simulink model "Teleoperation_Task_Space"  (R2021b)
settings: Solver=FixedStepAuto  StartTime=0.0  StopTime=20  FixedStep=Ts  RelTol=1e-3
values from neighbouring files (symbols this model uses):
  alphas_m = 25.0 * ones(1,dh.dof)    [setup_teleop.m]
  alphas_s = 16.5 * ones(1,dh.dof)    [setup_teleop.m]
  B_m = diag(ones(1,dh.dof)) * 32    [setup_teleop.m]
  B_s = diag(ones(1,dh.dof)) * 4    [setup_teleop.m]
  fc_in = 0.8    [setup_teleop.m]
  gravity = [0 0 9.81]'    [setup_robot.m]
  K_g = eye(dh.dof) * k_g    [setup_teleop.m]
  K_m = diag(ones(1,dh.dof)) * 22    [setup_teleop.m]
  K_s = diag(ones(1,dh.dof)) * 4    [setup_teleop.m]
  lambdas_m = 7.5 * ones(1,dh.dof)    [setup_teleop.m]
  lambdas_s = 3.0 * ones(1,dh.dof)    [setup_teleop.m]
  M_m = diag(ones(1,dh.dof)) * 22    [setup_teleop.m]
  M_s = diag(ones(1,dh.dof)) * 1    [setup_teleop.m]
  T_m2s = 25 / 1000 / Ts    (= 25)    [setup_teleop.m]
  T_s2m = 25 / 1000 / Ts    (= 25)    [setup_teleop.m]
  zdq_A = [1 3*wc 3*wc^2 wc^3]    [setup_teleop.m]
  zdq_B = [0 0 0 wc^3]    [setup_teleop.m]
undefined symbols (not defined in the file or in its folder): conf, dh, Fm_A, Fm_B, Fs_A, Fs_B, G, sigbuilder_block, x0
libraries: simulink x2, vrlib x2
(part 1 of 2)
settings Model: Creator=eros  LastModifiedBy=Sebastiano
settings SolverCC: AlgebraicLoopSolver=TrustRegion
settings DebuggingCC: SFMachineParentedDataDiag=warning

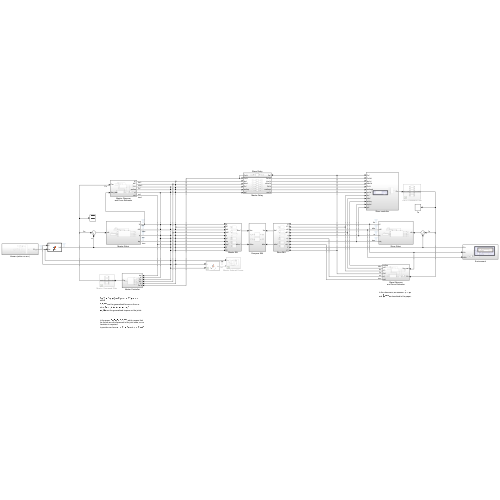
[thumbnail: Simulink's stored preview of the top-level diagram]
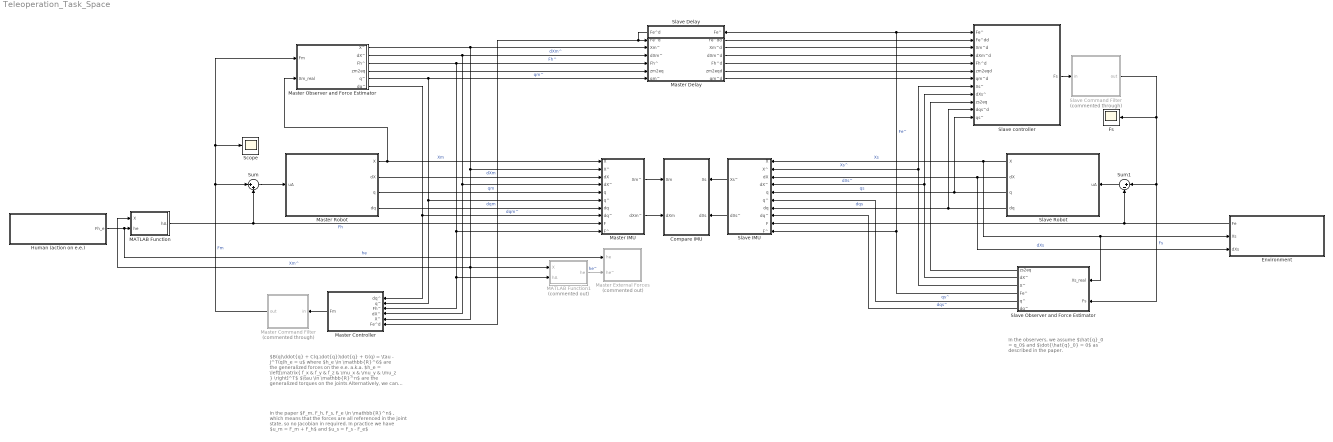
== system Teleoperation_Task_Space ==
  note: In the observers, we assume $\hat{q}_0 = q_0$ and $\dot{\hat{q}_0} = 0$ as described in the paper.
  note: In the paper $F_m, F_h, F_s, F_e \in \mathbb{R}^n$ , which means that the forces are all referenced in the joint state, so no Jacobian in required.
      | In practice we have $u_m = F_m + F_h$ and $u_s = F_s - F_e$
  note: $B(q)\ddot{q} + C(q,\dot{q})\dot{q} + G(q) = \tau - J^T(q)h_e = u$
      | where
      | $h_e \in \mathbb{R}^6$ are the generalized forces on the e.e.
      | a.k.a. $h_e = \left[\matrix{ f_x & f_y & f_z & \mu_x & \mu_y & \mu_z } \right]^T$
      | $\tau \in \mathbb{R}^n$ are the generalized torques on the joints
      |
      | Alternatively, we can write $\tau = J^T(q)\tau_e$ .
  Compare IMU : Subsystem
      settings: PortSchema="{\"entries\":[{\"content\":{\"sides\":[{\"content\":{\"connectorIds\":[\"In1\",\"In2\"]},\"type\":\"ConnectorPlacement.EquallySpacedRectSide\",\"uuid\":\"eee4eb85-6cb8-4462-85fc-1aafb3c3937f\"},{\"content\":{\"connectorIds\":[\"In3\",\"In4\"],\"side\":\"RIGHT\"},\"type\":\"ConnectorPlacement.EquallySpacedRectSide\",\"uuid\":\"5ab37ec6-6ee1-47e9-aff6-41baaee9b59b\"},{\"content\":{\"connectorIds\":[],\"side\":\"TOP\"},\"type\":\"ConnectorPlacement.EquallySpacedRectSide\",\"uuid\":\"6f11ee79-2d90-4b50-8360-b99d360f33b3\"}]},\"type\":\"ConnectorPlacement.EquallySpacedConnector\",\"uuid\":\"5676dc65-12f4-4a54-a0ce-a07c6c462ad2\"}],\"packageUris\":[\"http://schema.mathworks.com/mf0/Connector/R2020b\"],\"version\":\"1.0\"}"
  Environment : Subsystem
      settings: PortSchema="{\"entries\":[{\"content\":{\"sides\":[{\"content\":{\"connectorIds\":[\"Out1\",\"In1\",\"In2\"]},\"type\":\"ConnectorPlacement.EquallySpacedRectSide\",\"uuid\":\"3a683f5f-8229-405f-b97f-b506986b9524\"},{\"content\":{\"connectorIds\":[],\"side\":\"RIGHT\"},\"type\":\"ConnectorPlacement.EquallySpacedRectSide\",\"uuid\":\"ee737040-7d2a-42b5-b72e-c46d7dc1a0a9\"},{\"content\":{\"connectorIds\":[],\"side\":\"TOP\"},\"type\":\"ConnectorPlacement.EquallySpacedRectSide\",\"uuid\":\"297da6e9-ed01-499d-b3c2-0f0e3cad7b3e\"}]},\"type\":\"ConnectorPlacement.EquallySpacedConnector\",\"uuid\":\"c177a36f-944e-4ac9-b62c-2e9de2d24660\"}],\"packageUris\":[\"http://schema.mathworks.com/mf0/Connector/R2020b\"],\"version\":\"1.0\"}"
  Fs : Scope
  Human (action on e.e.) : Subsystem
  MATLAB Function : MATLAB Function  TreatAsAtomicUnit=on
  MATLAB Function1 : MATLAB Function  Commented=on  TreatAsAtomicUnit=on
  Master Command Filter : Subsystem  Commented=through
  Master Controller : Subsystem
  Master Delay : Subsystem
  Master External Forces : Subsystem  Commented=on
  Master IMU : Subsystem
  Master Observer and Force Estimator : Subsystem
  Master Robot : Subsystem
  Scope : Scope
  Slave Command Filter : Subsystem  Commented=through
  Slave Delay : Subsystem
  Slave IMU : Subsystem
  Slave Observer and Force Estimator : Subsystem
  Slave Robot : Subsystem
  Slave controller : Subsystem
  Sum : Sum  Inputs=|++
  Sum1 : Sum  Inputs=|+-
  wires:
  Slave Observer and Force Estimator/5(q^) -> Slave IMU/6(q^)  "qs^"
  Master Controller/1(Fm) -> Master Command Filter/1(in)
  Slave Observer and Force Estimator/1(zs2eq) -> Slave controller/10(zs2eq)
  Master Observer and Force Estimator/1(X^) -> Master Delay/2(Xm^), Master IMU/2(X^), MATLAB Function1/1(X), Master Controller/5(X^), MATLAB Function/1(X)  "Xm^"
  Slave Observer and Force Estimator/4(Fe^) -> Slave controller/1(Fe^), Slave Delay/1(Fe^), Slave IMU/10(F^)  "Fe^"
  Master Observer and Force Estimator/3(Fh^) -> Master Delay/4(Fh^), Master IMU/10(F^), MATLAB Function1/2(hA), Master Controller/3(Fh^)  "Fh^"
  Slave Observer and Force Estimator/6(dq^) -> Slave IMU/8(dq^)  "dqs^"
  Master Observer and Force Estimator/2(dX^) -> Master Delay/3(dXm^), Master IMU/4(dX^), Master Controller/4(dX^)  "dXm^"
  Slave controller/1(Fs) -> Slave Command Filter/1(in)
  Master Command Filter/1(out) -> Scope/1, Master Observer and Force Estimator/1(Fm), Sum/1  "Fm"
  Slave Command Filter/1(out) -> Slave Observer and Force Estimator/2(Fs), Sum1/1, Fs/1  "Fs"
  Master Observer and Force Estimator/4(zm2eq) -> Master Delay/5(zm2eq)
  Master Delay/1(Fe^dd) -> Slave controller/2(Fe^dd)
  Master Delay/3(dXm^d) -> Slave controller/4(dXm^d)
  Master Delay/2(Xm^d) -> Slave controller/3(Xm^d)
  Master Delay/4(Fh^d) -> Slave controller/5(Fh^d)
  Master Delay/5(zm2eqd) -> Slave controller/6(zm2eqd)
  Slave Delay/1(Fe^d) -> Master Controller/6(Fe^d), Master Delay/1(Fe^d)
  Slave Robot/3(q) -> Slave IMU/5(q), Slave controller/12(qs^)  "qs"
  Slave Robot/4(dq) -> Slave IMU/7(dq), Slave controller/11(dqs^d)  "dqs"
  MATLAB Function1/1(he) -> Master External Forces/2(he^)  "he^"
  Human (action on e.e.)/1(Fh_e) -> MATLAB Function/2(he), Master External Forces/1(he)  "he"
  Master Robot/1(X) -> Master Observer and Force Estimator/2(Xm_real), Master IMU/1(X)  "Xm"
  MATLAB Function/1(hA) -> Sum/2, Master IMU/9(F)  "Fh"
  Sum/1 -> Master Robot/1(uA)
  Master Robot/3(q) -> Master IMU/5(q)  "qm"
  Master Observer and Force Estimator/5(q^) -> Master Controller/2(q^), Master IMU/6(q^), Master Delay/6(qm^)  "qm^"
  Master Observer and Force Estimator/6(dq^) -> Master Controller/1(dq^), Master IMU/8(dq^)  "dqm^"
  Master Robot/4(dq) -> Master IMU/7(dq)  "dqm"
  Master Robot/2(dX) -> Master IMU/3(dX)  "dXm"
  Master IMU/2(dXm^) -> Compare IMU/2(dXm)
  Master IMU/1(Xm^) -> Compare IMU/1(Xm)
  Sum1/1 -> Slave Robot/1(uA)
  Slave Robot/1(X) -> Slave Observer and Force Estimator/1(Xs_real), Environment/1(Xs), Slave IMU/1(X)  "Xs"
  Slave Robot/2(dX) -> Environment/2(dXs), Slave IMU/3(dX)  "dXs"
  Slave Observer and Force Estimator/3(X^) -> Slave controller/8(Xs^), Slave IMU/2(X^)  "Xs^"
  Slave Observer and Force Estimator/2(dX^) -> Slave IMU/4(dX^), Slave controller/9(dXs^)  "dXs^"
  Slave IMU/1(Xs^) -> Compare IMU/3(Xs)
  Slave IMU/2(dXs^) -> Compare IMU/4(dXs)
  Master Delay/6(qm^d) -> Slave controller/7(qm^d)
  Environment/1(Fe) -> Sum1/2, Slave IMU/9(F)

== system Teleoperation_Task_Space/Compare IMU ==
  Xm : Inport
  dXm : Inport  Port=2
  Xs : Inport  Port=3
  dXs : Inport  Port=4
  Speed : Subsystem
      settings: PortSchema="{\"entries\":[{\"content\":{\"sides\":[{\"content\":{\"connectorIds\":[\"In1\"]},\"type\":\"ConnectorPlacement.EquallySpacedRectSide\",\"uuid\":\"98f8c5d8-e26e-427c-a81e-60bbe3a3ab4d\"},{\"content\":{\"connectorIds\":[\"In2\"],\"side\":\"RIGHT\"},\"type\":\"ConnectorPlacement.EquallySpacedRectSide\",\"uuid\":\"a51aa647-09cd-4fb3-b31a-f2bc2bc6e0ff\"},{\"content\":{\"connectorIds\":[],\"side\":\"TOP\"},\"type\":\"ConnectorPlacement.EquallySpacedRectSide\",\"uuid\":\"9387bbe5-2fda-43cb-b346-55f243092f42\"}]},\"type\":\"ConnectorPlacement.EquallySpacedConnector\",\"uuid\":\"8debe184-3b59-4f16-84f4-2d6030e17ba5\"}],\"packageUris\":[\"http://schema.mathworks.com/mf0/Connector/R2020b\"],\"version\":\"1.0\"}"
  State : Subsystem
      settings: PortSchema="{\"entries\":[{\"content\":{\"sides\":[{\"content\":{\"connectorIds\":[\"In1\"]},\"type\":\"ConnectorPlacement.EquallySpacedRectSide\",\"uuid\":\"98f8c5d8-e26e-427c-a81e-60bbe3a3ab4d\"},{\"content\":{\"connectorIds\":[\"In2\"],\"side\":\"RIGHT\"},\"type\":\"ConnectorPlacement.EquallySpacedRectSide\",\"uuid\":\"a51aa647-09cd-4fb3-b31a-f2bc2bc6e0ff\"},{\"content\":{\"connectorIds\":[],\"side\":\"TOP\"},\"type\":\"ConnectorPlacement.EquallySpacedRectSide\",\"uuid\":\"9387bbe5-2fda-43cb-b346-55f243092f42\"}]},\"type\":\"ConnectorPlacement.EquallySpacedConnector\",\"uuid\":\"8debe184-3b59-4f16-84f4-2d6030e17ba5\"}],\"packageUris\":[\"http://schema.mathworks.com/mf0/Connector/R2020b\"],\"version\":\"1.0\"}"
  wires:
  Xm/1 -> State/2(q_m)
  Xs/1 -> State/1(q_s)
  dXm/1 -> Speed/1(dq_m)
  dXs/1 -> Speed/2(dq_s)

== system Teleoperation_Task_Space/Environment ==
  note: Spring Environment
  note: Spring-Damper Environment
  Xs : Inport
  dXs : Inport  Port=2
  Constant1 : Constant  Value=[0 0]
  Constant2 : Constant  Value=[0.43 0.41]
  Constant3 : Constant  Value=[0 0]
  Manual Switch : ManualSwitch
  Manual Switch1 : ManualSwitch
  Multiply : Gain  Gain=150*eye(2)  Multiplication=Matrix(K*u)
  Multiply1 : Gain  Gain=10*eye(2)  Multiplication=Matrix(K*u)
  Sum : Sum  Inputs=|++
  Sum2 : Sum  Inputs=+-|
  Fe : Outport
  wires:
  Sum/1 -> Manual Switch/1
  Sum2/1 -> Multiply/1
  Constant2/1 -> Sum2/2
  Xs/1 -> Sum2/1
  Constant1/1 -> Manual Switch1/2
  Manual Switch/1 -> Fe/1
  Multiply/1 -> Sum/1
  Manual Switch1/1 -> Sum/2
  Multiply1/1 -> Manual Switch1/1
  dXs/1 -> Multiply1/1
  Constant3/1 -> Manual Switch/2

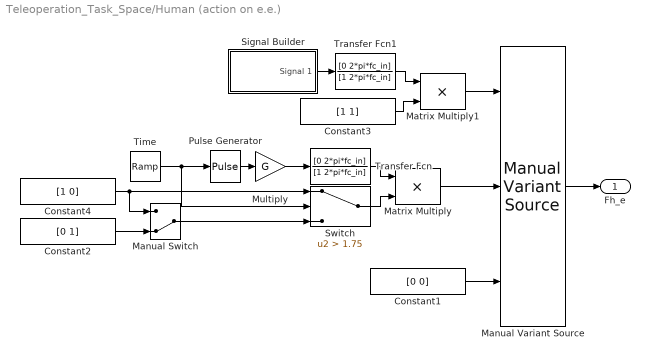
== system Teleoperation_Task_Space/Human (action on e.e.) ==
  Constant1 : Constant  Value=[0 0]
  Constant2 : Constant  Value=[0 1]
  Constant3 : Constant  Value=[1 1]
  Constant4 : Constant  Value=[1 0]
  Manual Variant Source : simulink/Signal Routing/Manual Variant Source  NumChoices=3  LabelModeActiveChoice=V_1
  Manual Switch : ManualSwitch  CurrentSetting=0
  Matrix Multiply : Product
  Matrix Multiply1 : Product
  Multiply : Gain  Gain=G
  Pulse Generator : DiscretePulseGenerator  PulseType=Time based  TimeSource=Use external signal  Period=10  PulseWidth=5  PhaseDelay=0.5
  Signal Builder : Subsystem  Tag=STV Subsys  LoadFcn=sigbuilder_block('load');  StartFcn=sigbuilder_block('start');  StopFcn=sigbuilder_block('stop');  ClipboardFcn=sigbuilder_block('clipboard');  mask(Sigbuilder block){tuvar=[0:10]}
      mask help: Simulink:masks:SigbuilderBlock_MD
      mask init:
      | if ~strcmp(get_param(bdroot(gcbh),'SimulationStatus'),'stopped') tuvar = sigbuilder_block('maskInit'); end
      settings: CopyFcn=sigbuilder_block('copy');  DeleteFcn=sigbuilder_block('delete');  ModelCloseFcn=sigbuilder_block('modelClose');  PreSaveFcn=sigbuilder_block('preSave');  PauseFcn=sigbuilder_block('pause');  ContinueFcn=sigbuilder_block('continue');  NameChangeFcn=sigbuilder_block('namechange');  OpenFcn=sigbuilder_block('open',[47.25 0 1392.75 752.25 ]);  CloseFcn=sigbuilder_block('close');
      mask Display: plot(0, 0, 100, 100,[2, 2, 32, 32, 2], [68, 8, 8, 68, 68],[32, 2], [38, 38], [32, 19, 2],[53, 60, 44], [32, 17, 17, 2],[16, 16, 31, 31]);txt = getActiveGroup(gcbh);text(2, 100, txt,'verticalAlignment', 'top');
  Switch : Switch  Criteria=u2 > Threshold  Threshold=1.75
  Time : simulink/Sources/Ramp  slope=1  start=0  InitialOutput=0
  Transfer Fcn : TransferFcn  Numerator=[0 2*pi*fc_in]  Denominator=[1 2*pi*fc_in]
  Transfer Fcn1 : TransferFcn  Numerator=[0 2*pi*fc_in]  Denominator=[1 2*pi*fc_in]
  Fh_e : Outport
  wires:
  Switch/1 -> Matrix Multiply/2
  Constant2/1 -> Manual Switch/2
  Transfer Fcn/1 -> Matrix Multiply/1
  Time/1 -> Switch/2, Pulse Generator/1
  Constant4/1 -> Manual Switch/1, Switch/1
  Manual Switch/1 -> Switch/3
  Matrix Multiply/1 -> Manual Variant Source/2
  Constant1/1 -> Manual Variant Source/3
  Signal Builder/1(Signal 1) -> Transfer Fcn1/1
  Pulse Generator/1 -> Multiply/1
  Multiply/1 -> Transfer Fcn/1
  Transfer Fcn1/1 -> Matrix Multiply1/1
  Constant3/1 -> Matrix Multiply1/2
  Matrix Multiply1/1 -> Manual Variant Source/1
  Manual Variant Source/1 -> Fh_e/1

== system Teleoperation_Task_Space/Master Command Filter ==
  in : Inport
  Demux : Demux  Outputs=6
  Filter{,1..5} (6 alike) : TransferFcn  Numerator=Fm_B  Denominator=Fm_A
  Mux : Mux  Inputs=6
  out : Outport
  wires:
  Demux/4 -> Filter3/1
  Demux/6 -> Filter5/1
  Demux/2 -> Filter1/1
  Demux/5 -> Filter4/1
  Demux/1 -> Filter/1
  Demux/3 -> Filter2/1
  in/1 -> Demux/1
  Mux/1 -> out/1
  Filter/1 -> Mux/1
  Filter1/1 -> Mux/2
  Filter2/1 -> Mux/3
  Filter3/1 -> Mux/4
  Filter4/1 -> Mux/5
  Filter5/1 -> Mux/6

== system Teleoperation_Task_Space/Master Controller ==
  note: Here we provide q^ and dq^ just to avoid calculating them
  dq^ : Inport
  q^ : Inport  Port=2
  Fh^ : Inport  Port=3
  dX^ : Inport  Port=4
  X^ : Inport  Port=5
  Fe^d : Inport  Port=6
  Master Controller : MATLAB Function  TreatAsAtomicUnit=on
  Fm : Outport
  wires:
  Fh^/1 -> Master Controller/5(Fh)
  Fe^d/1 -> Master Controller/6(Fe_d)
  Master Controller/1(Fm) -> Fm/1  "Fm"
  X^/1 -> Master Controller/3(Xm)
  dX^/1 -> Master Controller/4(dXm)
  dq^/1 -> Master Controller/2(dqm)
  q^/1 -> Master Controller/1(qm)

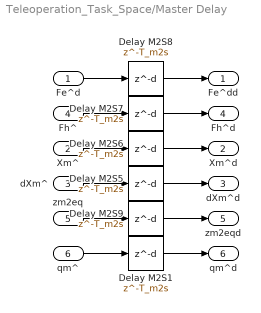
== system Teleoperation_Task_Space/Master Delay ==
  Fe^d : Inport
  Xm^ : Inport  Port=2
  dXm^ : Inport  Port=3
  Fh^ : Inport  Port=4
  zm2eq : Inport  Port=5
  qm^ : Inport  Port=6
  Delay M2S{1,5..9} (6 alike) : Delay  DelayLength=T_m2s
  Fe^dd : Outport
  Xm^d : Outport  Port=2
  dXm^d : Outport  Port=3
  Fh^d : Outport  Port=4
  zm2eqd : Outport  Port=5
  qm^d : Outport  Port=6
  wires:
  zm2eq/1 -> Delay M2S9/1
  Delay M2S6/1 -> Xm^d/1
  dXm^/1 -> Delay M2S5/1
  Fe^d/1 -> Delay M2S8/1
  Fh^/1 -> Delay M2S7/1
  Delay M2S5/1 -> dXm^d/1
  Delay M2S7/1 -> Fh^d/1
  Xm^/1 -> Delay M2S6/1
  Delay M2S8/1 -> Fe^dd/1
  Delay M2S9/1 -> zm2eqd/1
  Delay M2S1/1 -> qm^d/1
  qm^/1 -> Delay M2S1/1

== system Teleoperation_Task_Space/Master External Forces ==
  he : Inport
  he^ : Inport  Port=2
  Master he : Scope  NumInputPorts=2
  Mux : Mux  Inputs=2
  Mux1 : Mux  Inputs=2
  qm : Demux  Outputs=dh.dof
  qs : Demux  Outputs=dh.dof
  wires:
  he/1 -> qm/1
  he^/1 -> qs/1
  qm/1 -> Mux/1
  qs/1 -> Mux/2
  qm/2 -> Mux1/1
  qs/2 -> Mux1/2
  Mux/1 -> Master he/1
  Mux1/1 -> Master he/2

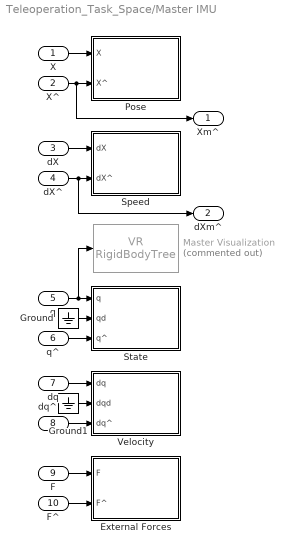
== system Teleoperation_Task_Space/Master IMU ==
  X : Inport
  X^ : Inport  Port=2
  dX : Inport  Port=3
  dX^ : Inport  Port=4
  q : Inport  Port=5
  q^ : Inport  Port=6
  dq : Inport  Port=7
  dq^ : Inport  Port=8
  F : Inport  Port=9
  F^ : Inport  Port=10
  External Forces : Subsystem
  Ground : Ground
  Ground1 : Ground
  Master Visualization : vrlib/VR RigidBodyTree  Commented=on  RBT=UR5_robot  useRBT=on  Ts=-1  ForceViewerOpen=on
      settings: SourceProductBaseCode=SL
  Pose : Subsystem
  Speed : Subsystem
  State : Subsystem
  Velocity : Subsystem
  Xm^ : Outport
  dXm^ : Outport  Port=2
  wires:
  q/1 -> Master Visualization/1, State/1(q)
  q^/1 -> State/3(q^)
  F/1 -> External Forces/1(F)
  dq/1 -> Velocity/1(dq)
  F^/1 -> External Forces/2(F^)
  dq^/1 -> Velocity/3(dq^)
  Ground/1 -> State/2(qd)
  Ground1/1 -> Velocity/2(dqd)
  X^/1 -> Xm^/1, Pose/2(X^)
  X/1 -> Pose/1(X)
  dX/1 -> Speed/1(dX)
  dX^/1 -> dXm^/1, Speed/2(dX^)

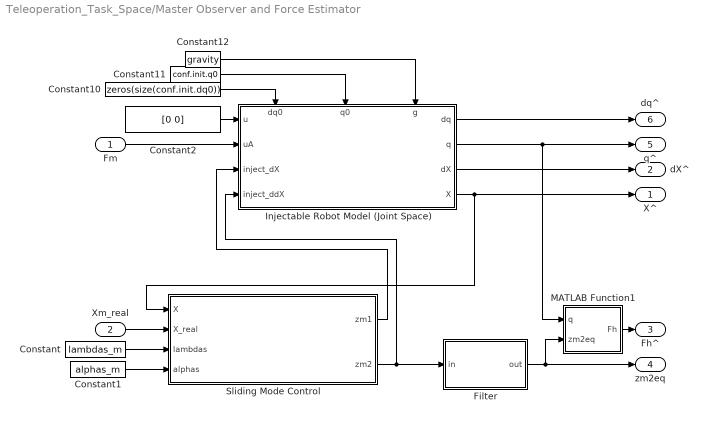
== system Teleoperation_Task_Space/Master Observer and Force Estimator ==
  Fm : Inport
  Xm_real : Inport  Port=2
  Constant : Constant  Value=lambdas_m
  Constant1 : Constant  Value=alphas_m
  Constant10 : Constant  Value=zeros(size(conf.init.dq0))
  Constant11 : Constant  Value=conf.init.q0
  Constant12 : Constant  Value=gravity
  Constant2 : Constant  Value=[0 0]
  Filter : Subsystem
  Injectable Robot Model (Joint Space) : Subsystem
      settings: PortSchema="{\"entries\":[{\"content\":{\"sides\":[{\"content\":{\"connectorIds\":[\"In1\",\"In2\",\"In3\",\"In4\"]},\"type\":\"ConnectorPlacement.EquallySpacedRectSide\",\"uuid\":\"a8701c64-329e-4144-b882-ecf5d621aff2\"},{\"content\":{\"connectorIds\":[\"Out1\",\"Out2\",\"Out3\",\"Out4\"],\"side\":\"RIGHT\"},\"type\":\"ConnectorPlacement.EquallySpacedRectSide\",\"uuid\":\"4e168703-1cb9-438c-bc6b-9b2d7fbb809e\"},{\"content\":{\"connectorIds\":[\"In5\",\"In6\",\"In7\"],\"side\":\"TOP\"},\"type\":\"ConnectorPlacement.EquallySpacedRectSide\",\"uuid\":\"8fbcb29e-7fab-4224-b4ad-ee01c13d675a\"}]},\"type\":\"ConnectorPlacement.EquallySpacedConnector\",\"uuid\":\"fa721fab-1ce6-4fdf-95fa-8ada3ed2d65c\"}],\"packageUris\":[\"http://schema.mathworks.com/mf0/Connector/R2020b\"],\"version\":\"1.0\"}"
  MATLAB Function1 : MATLAB Function  TreatAsAtomicUnit=on
  Sliding Mode Control : Subsystem
  X^ : Outport
  dX^ : Outport  Port=2
  Fh^ : Outport  Port=3
  zm2eq : Outport  Port=4
  q^ : Outport  Port=5
  dq^ : Outport  Port=6
  wires:
  Filter/1(out) -> MATLAB Function1/2(zm2eq), zm2eq/1
  Sliding Mode Control/1(zm1) -> Injectable Robot Model (Joint Space)/3(inject_dX)
  Sliding Mode Control/2(zm2) -> Injectable Robot Model (Joint Space)/4(inject_ddX), Filter/1(in)
  Constant1/1 -> Sliding Mode Control/4(alphas)
  Constant/1 -> Sliding Mode Control/3(lambdas)
  Xm_real/1 -> Sliding Mode Control/2(X_real)
  Injectable Robot Model (Joint Space)/4(X) -> X^/1, Sliding Mode Control/1(X)
  Injectable Robot Model (Joint Space)/3(dX) -> dX^/1
  Constant11/1 -> Injectable Robot Model (Joint Space)/6(q0)
  Constant10/1 -> Injectable Robot Model (Joint Space)/5(dq0)
  Injectable Robot Model (Joint Space)/1(dq) -> dq^/1
  Constant12/1 -> Injectable Robot Model (Joint Space)/7(g)
  Injectable Robot Model (Joint Space)/2(q) -> MATLAB Function1/1(q), q^/1
  MATLAB Function1/1(Fh) -> Fh^/1
  Constant2/1 -> Injectable Robot Model (Joint Space)/1(u)
  Fm/1 -> Injectable Robot Model (Joint Space)/2(uA)

== system Teleoperation_Task_Space/Master Robot ==
  uA : Inport
  Constant10 : Constant  Value=conf.init.dq0
  Constant11 : Constant  Value=conf.init.q0
  Constant12 : Constant  Value=gravity
  Constant3 : Constant  Value=[0 0]
  Injectable Robot Model (Joint Space) : Subsystem
      settings: PortSchema="{\"entries\":[{\"content\":{\"sides\":[{\"content\":{\"connectorIds\":[\"In1\",\"In2\",\"In3\",\"In4\"]},\"type\":\"ConnectorPlacement.EquallySpacedRectSide\",\"uuid\":\"a8701c64-329e-4144-b882-ecf5d621aff2\"},{\"content\":{\"connectorIds\":[\"Out1\",\"Out2\",\"Out3\",\"Out4\"],\"side\":\"RIGHT\"},\"type\":\"ConnectorPlacement.EquallySpacedRectSide\",\"uuid\":\"4e168703-1cb9-438c-bc6b-9b2d7fbb809e\"},{\"content\":{\"connectorIds\":[\"In5\",\"In6\",\"In7\"],\"side\":\"TOP\"},\"type\":\"ConnectorPlacement.EquallySpacedRectSide\",\"uuid\":\"8fbcb29e-7fab-4224-b4ad-ee01c13d675a\"}]},\"type\":\"ConnectorPlacement.EquallySpacedConnector\",\"uuid\":\"fa721fab-1ce6-4fdf-95fa-8ada3ed2d65c\"}],\"packageUris\":[\"http://schema.mathworks.com/mf0/Connector/R2020b\"],\"version\":\"1.0\"}"
  X : Outport
  dX : Outport  Port=2
  q : Outport  Port=3
  dq : Outport  Port=4
  wires:
  Constant10/1 -> Injectable Robot Model (Joint Space)/5(dq0)
  Constant3/1 -> Injectable Robot Model (Joint Space)/1(u), Injectable Robot Model (Joint Space)/4(inject_ddX), Injectable Robot Model (Joint Space)/3(inject_dX)
  Constant11/1 -> Injectable Robot Model (Joint Space)/6(q0)
  Injectable Robot Model (Joint Space)/2(q) -> q/1
  Injectable Robot Model (Joint Space)/3(dX) -> dX/1
  Constant12/1 -> Injectable Robot Model (Joint Space)/7(g)
  Injectable Robot Model (Joint Space)/4(X) -> X/1
  Injectable Robot Model (Joint Space)/1(dq) -> dq/1
  uA/1 -> Injectable Robot Model (Joint Space)/2(uA)

== system Teleoperation_Task_Space/Slave Command Filter ==
  in : Inport
  Demux : Demux  Outputs=6
  Filter{,1..5} (6 alike) : TransferFcn  Numerator=Fs_B  Denominator=Fs_A
  Mux : Mux  Inputs=6
  out : Outport
  wires:
  Demux/4 -> Filter3/1
  Demux/6 -> Filter5/1
  Demux/2 -> Filter1/1
  Demux/5 -> Filter4/1
  Demux/1 -> Filter/1
  Demux/3 -> Filter2/1
  in/1 -> Demux/1
  Mux/1 -> out/1
  Filter/1 -> Mux/1
  Filter2/1 -> Mux/3
  Filter3/1 -> Mux/4
  Filter4/1 -> Mux/5
  Filter5/1 -> Mux/6
  Filter1/1 -> Mux/2

== system Teleoperation_Task_Space/Slave Delay ==
  Fe^ : Inport
  Delay S2M1 : Delay  DelayLength=T_s2m
  Fe^d : Outport
  wires:
  Delay S2M1/1 -> Fe^d/1
  Fe^/1 -> Delay S2M1/1

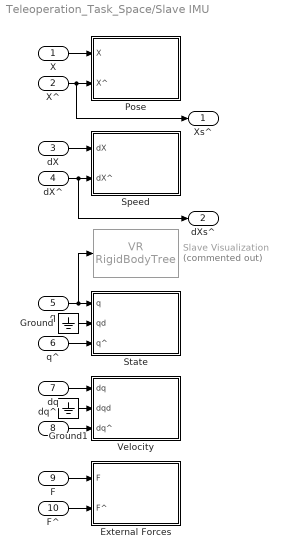
== system Teleoperation_Task_Space/Slave IMU ==
  X : Inport
  X^ : Inport  Port=2
  dX : Inport  Port=3
  dX^ : Inport  Port=4
  q : Inport  Port=5
  q^ : Inport  Port=6
  dq : Inport  Port=7
  dq^ : Inport  Port=8
  F : Inport  Port=9
  F^ : Inport  Port=10
  External Forces : Subsystem
  Ground : Ground
  Ground1 : Ground
  Pose : Subsystem
  Slave Visualization : vrlib/VR RigidBodyTree  Commented=on  RBT=UR5_robot  useRBT=on  Ts=-1  ForceViewerOpen=on
      settings: SourceProductBaseCode=SL
  Speed : Subsystem
  State : Subsystem
  Velocity : Subsystem
  Xs^ : Outport
  dXs^ : Outport  Port=2
  wires:
  q/1 -> Slave Visualization/1, State/1(q)
  q^/1 -> State/3(q^)
  F/1 -> External Forces/1(F)
  dq/1 -> Velocity/1(dq)
  F^/1 -> External Forces/2(F^)
  dq^/1 -> Velocity/3(dq^)
  Ground/1 -> State/2(qd)
  Ground1/1 -> Velocity/2(dqd)
  X^/1 -> Xs^/1, Pose/2(X^)
  X/1 -> Pose/1(X)
  dX/1 -> Speed/1(dX)
  dX^/1 -> dXs^/1, Speed/2(dX^)

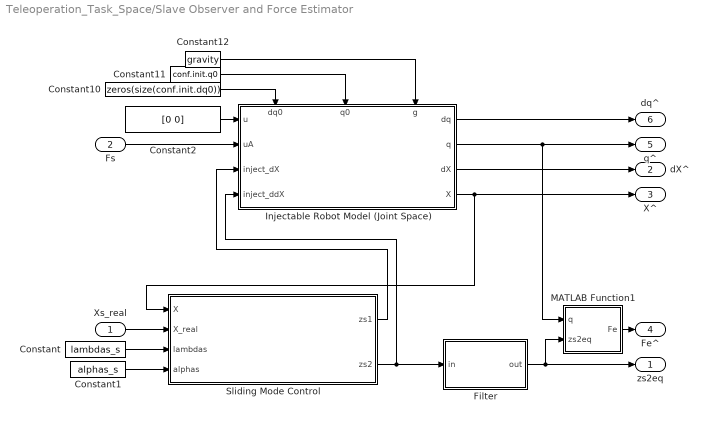
== system Teleoperation_Task_Space/Slave Observer and Force Estimator ==
  Xs_real : Inport
  Fs : Inport  Port=2
  Constant : Constant  Value=lambdas_s
  Constant1 : Constant  Value=alphas_s
  Constant10 : Constant  Value=zeros(size(conf.init.dq0))
  Constant11 : Constant  Value=conf.init.q0
  Constant12 : Constant  Value=gravity
  Constant2 : Constant  Value=[0 0]
  Filter : Subsystem
  Injectable Robot Model (Joint Space) : Subsystem
      settings: PortSchema="{\"entries\":[{\"content\":{\"sides\":[{\"content\":{\"connectorIds\":[\"In1\",\"In2\",\"In3\",\"In4\"]},\"type\":\"ConnectorPlacement.EquallySpacedRectSide\",\"uuid\":\"a8701c64-329e-4144-b882-ecf5d621aff2\"},{\"content\":{\"connectorIds\":[\"Out1\",\"Out2\",\"Out3\",\"Out4\"],\"side\":\"RIGHT\"},\"type\":\"ConnectorPlacement.EquallySpacedRectSide\",\"uuid\":\"4e168703-1cb9-438c-bc6b-9b2d7fbb809e\"},{\"content\":{\"connectorIds\":[\"In5\",\"In6\",\"In7\"],\"side\":\"TOP\"},\"type\":\"ConnectorPlacement.EquallySpacedRectSide\",\"uuid\":\"8fbcb29e-7fab-4224-b4ad-ee01c13d675a\"}]},\"type\":\"ConnectorPlacement.EquallySpacedConnector\",\"uuid\":\"fa721fab-1ce6-4fdf-95fa-8ada3ed2d65c\"}],\"packageUris\":[\"http://schema.mathworks.com/mf0/Connector/R2020b\"],\"version\":\"1.0\"}"
  MATLAB Function1 : MATLAB Function  TreatAsAtomicUnit=on
  Sliding Mode Control : Subsystem
  zs2eq : Outport
  dX^ : Outport  Port=2
  X^ : Outport  Port=3
  Fe^ : Outport  Port=4
  q^ : Outport  Port=5
  dq^ : Outport  Port=6
  wires:
  Filter/1(out) -> MATLAB Function1/2(zs2eq), zs2eq/1
  Sliding Mode Control/1(zs1) -> Injectable Robot Model (Joint Space)/3(inject_dX)
  Sliding Mode Control/2(zs2) -> Injectable Robot Model (Joint Space)/4(inject_ddX), Filter/1(in)
  Constant1/1 -> Sliding Mode Control/4(alphas)
  Constant/1 -> Sliding Mode Control/3(lambdas)
  Xs_real/1 -> Sliding Mode Control/2(X_real)
  Injectable Robot Model (Joint Space)/4(X) -> X^/1, Sliding Mode Control/1(X)
  Injectable Robot Model (Joint Space)/3(dX) -> dX^/1
  Constant11/1 -> Injectable Robot Model (Joint Space)/6(q0)
  Constant10/1 -> Injectable Robot Model (Joint Space)/5(dq0)
  Injectable Robot Model (Joint Space)/1(dq) -> dq^/1
  Constant12/1 -> Injectable Robot Model (Joint Space)/7(g)
  Injectable Robot Model (Joint Space)/2(q) -> MATLAB Function1/1(q), q^/1
  MATLAB Function1/1(Fe) -> Fe^/1
  Constant2/1 -> Injectable Robot Model (Joint Space)/1(u)
  Fs/1 -> Injectable Robot Model (Joint Space)/2(uA)

== system Teleoperation_Task_Space/Slave Robot ==
  uA : Inport
  Constant10 : Constant  Value=conf.init.dq0
  Constant11 : Constant  Value=conf.init.q0
  Constant12 : Constant  Value=gravity
  Constant3 : Constant  Value=[0 0]
  Injectable Robot Model (Joint Space) : Subsystem
      settings: PortSchema="{\"entries\":[{\"content\":{\"sides\":[{\"content\":{\"connectorIds\":[\"In1\",\"In2\",\"In3\",\"In4\"]},\"type\":\"ConnectorPlacement.EquallySpacedRectSide\",\"uuid\":\"a8701c64-329e-4144-b882-ecf5d621aff2\"},{\"content\":{\"connectorIds\":[\"Out1\",\"Out2\",\"Out3\",\"Out4\"],\"side\":\"RIGHT\"},\"type\":\"ConnectorPlacement.EquallySpacedRectSide\",\"uuid\":\"4e168703-1cb9-438c-bc6b-9b2d7fbb809e\"},{\"content\":{\"connectorIds\":[\"In5\",\"In6\",\"In7\"],\"side\":\"TOP\"},\"type\":\"ConnectorPlacement.EquallySpacedRectSide\",\"uuid\":\"8fbcb29e-7fab-4224-b4ad-ee01c13d675a\"}]},\"type\":\"ConnectorPlacement.EquallySpacedConnector\",\"uuid\":\"fa721fab-1ce6-4fdf-95fa-8ada3ed2d65c\"}],\"packageUris\":[\"http://schema.mathworks.com/mf0/Connector/R2020b\"],\"version\":\"1.0\"}"
  X : Outport
  dX : Outport  Port=2
  q : Outport  Port=3
  dq : Outport  Port=4
  wires:
  Constant10/1 -> Injectable Robot Model (Joint Space)/5(dq0)
  Constant3/1 -> Injectable Robot Model (Joint Space)/1(u), Injectable Robot Model (Joint Space)/4(inject_ddX), Injectable Robot Model (Joint Space)/3(inject_dX)
  Constant11/1 -> Injectable Robot Model (Joint Space)/6(q0)
  Injectable Robot Model (Joint Space)/2(q) -> q/1
  Injectable Robot Model (Joint Space)/3(dX) -> dX/1
  Constant12/1 -> Injectable Robot Model (Joint Space)/7(g)
  Injectable Robot Model (Joint Space)/4(X) -> X/1
  Injectable Robot Model (Joint Space)/1(dq) -> dq/1
  uA/1 -> Injectable Robot Model (Joint Space)/2(uA)

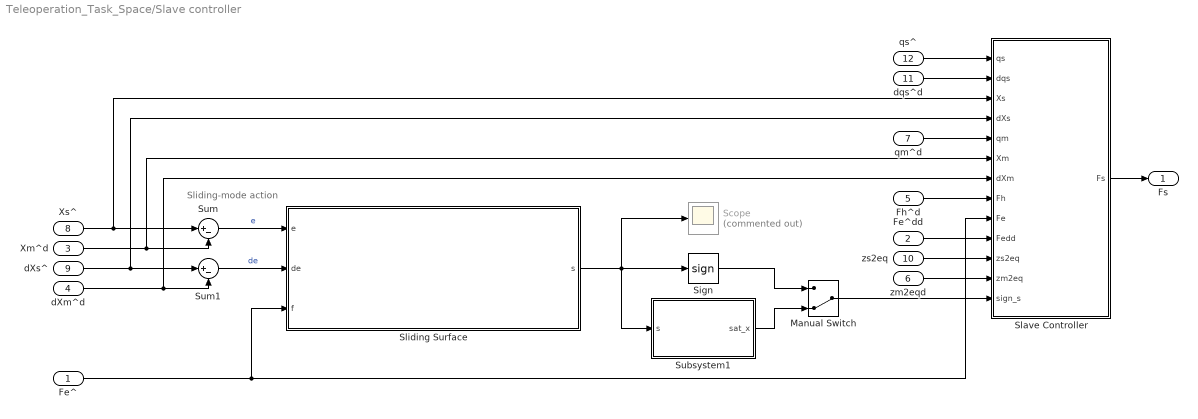
== system Teleoperation_Task_Space/Slave controller ==
  note: Sliding-mode action
  Fe^ : Inport
  Fe^dd : Inport  Port=2
  Xm^d : Inport  Port=3
  dXm^d : Inport  Port=4
  Fh^d : Inport  Port=5
  zm2eqd : Inport  Port=6
  qm^d : Inport  Port=7
  Xs^ : Inport  Port=8
  dXs^ : Inport  Port=9
  zs2eq : Inport  Port=10
  dqs^d : Inport  Port=11
  qs^ : Inport  Port=12
  Manual Switch : ManualSwitch  CurrentSetting=0
  Scope : Scope  Commented=on
  Sign : Signum
  Slave Controller : MATLAB Function  TreatAsAtomicUnit=on
  Sliding Surface : Subsystem
  Subsystem1 : Subsystem
  Sum : Sum  Inputs=|+-
  Sum1 : Sum  Inputs=|+-
  Fs : Outport
  wires:
  zs2eq/1 -> Slave Controller/11(zs2eq)
  Fh^d/1 -> Slave Controller/8(Fh)
  Slave Controller/1(Fs) -> Fs/1
  zm2eqd/1 -> Slave Controller/12(zm2eq)
  Fe^dd/1 -> Slave Controller/10(Fedd)
  Xs^/1 -> Sum/1, Slave Controller/3(Xs)
  Xm^d/1 -> Sum/2, Slave Controller/6(Xm)
  dXs^/1 -> Sum1/1, Slave Controller/4(dXs)
  dXm^d/1 -> Slave Controller/7(dXm), Sum1/2
  Fe^/1 -> Slave Controller/9(Fe), Sliding Surface/3(f)
  Sign/1 -> Manual Switch/1
  Sum/1 -> Sliding Surface/1(e)  "e"
  Sum1/1 -> Sliding Surface/2(de)  "de"
  Sliding Surface/1(s) -> Sign/1, Scope/1, Subsystem1/1(s)
  Subsystem1/1(sat_x) -> Manual Switch/2
  Manual Switch/1 -> Slave Controller/13(sign_s)
  qs^/1 -> Slave Controller/1(qs)
  dqs^d/1 -> Slave Controller/2(dqs)
  qm^d/1 -> Slave Controller/5(qm)

== system Teleoperation_Task_Space/Compare IMU/Speed ==
  dq_m : Inport
  dq_s : Inport  Port=2
  Compare Speed : Scope  NumInputPorts=2
  Mux : Mux  Inputs=2
  Mux1 : Mux  Inputs=2
  qm : Demux  Outputs=dh.dof
  qs : Demux  Outputs=dh.dof
  wires:
  dq_m/1 -> qm/1
  dq_s/1 -> qs/1
  qm/1 -> Mux/1
  qs/1 -> Mux/2
  qm/2 -> Mux1/1
  qs/2 -> Mux1/2
  Mux/1 -> Compare Speed/1
  Mux1/1 -> Compare Speed/2

== system Teleoperation_Task_Space/Compare IMU/State ==
  q_s : Inport
  q_m : Inport  Port=2
  Compare State : Scope  NumInputPorts=2
  Mux : Mux  Inputs=2
  Mux1 : Mux  Inputs=2
  qm : Demux  Outputs=dh.dof
  qs : Demux  Outputs=dh.dof
  wires:
  q_m/1 -> qm/1
  q_s/1 -> qs/1
  qm/1 -> Mux/1
  qs/1 -> Mux/2
  qm/2 -> Mux1/1
  qs/2 -> Mux1/2
  Mux/1 -> Compare State/1
  Mux1/1 -> Compare State/2

== system Teleoperation_Task_Space/Human (action on e.e.)/Signal Builder ==
  Demux : Demux  Tag=STV Demux  Outputs=1
      settings: DisplayOption=none
  FromWs : FromWorkspace  Tag=STV FromWs  VariableName=tuvar
      SigBuilderData=|
      | common.afterFinalStr = 'Extrapolate'
      | common.sampleTime = 0
      | dataSet.timeRange = [0 20]
      | dataSet.name = 'Group 1'
      | sbobj.Groups.Name = 'Group 1'
      | sbobj.Groups.Signals.Name = 'Signal 1'
      | sbobj.Groups.Signals.XData = [0 5 5 10 10 15 15 20]
      | sbobj.Groups.Signals.YData = [10 10 5 5 10 10 5 5]
      | sbobj.Groups.TimeRange = [0 20]
  Signal 1 : Outport  Tag=STV Outport
  wires:
  Demux/1 -> Signal 1/1
  FromWs/1 -> Demux/1

== system Teleoperation_Task_Space/Master IMU/External Forces ==
  F : Inport
  F^ : Inport  Port=2
  Master Fe : Scope  NumInputPorts=2
  Mux : Mux  Inputs=2
  Mux1 : Mux  Inputs=2
  qm : Demux  Outputs=dh.dof
  qs : Demux  Outputs=dh.dof
  wires:
  F/1 -> qm/1
  F^/1 -> qs/1
  qm/1 -> Mux/1
  qs/1 -> Mux/2
  qm/2 -> Mux1/1
  qs/2 -> Mux1/2
  Mux/1 -> Master Fe/1
  Mux1/1 -> Master Fe/2

== system Teleoperation_Task_Space/Master IMU/Pose ==
  X : Inport
  X^ : Inport  Port=2
  Master Pose : Scope  NumInputPorts=2
  Mux : Mux  Inputs=2
  Mux1 : Mux  Inputs=2
  qm : Demux  Outputs=dh.dof
  qm1 : Demux  Outputs=dh.dof
  wires:
  X/1 -> qm/1
  qm/1 -> Mux/1
  qm/2 -> Mux1/1
  Mux/1 -> Master Pose/1
  Mux1/1 -> Master Pose/2
  qm1/2 -> Mux1/2
  X^/1 -> qm1/1
  qm1/1 -> Mux/2

== system Teleoperation_Task_Space/Master IMU/Speed ==
  dX : Inport
  dX^ : Inport  Port=2
  Master Speed : Scope  NumInputPorts=2
  Mux : Mux  Inputs=2
  Mux1 : Mux  Inputs=2
  qm : Demux  Outputs=dh.dof
  qm1 : Demux  Outputs=dh.dof
  wires:
  dX/1 -> qm/1
  qm/1 -> Mux/1
  qm/2 -> Mux1/1
  Mux/1 -> Master Speed/1
  Mux1/1 -> Master Speed/2
  qm1/2 -> Mux1/2
  dX^/1 -> qm1/1
  qm1/1 -> Mux/2

== system Teleoperation_Task_Space/Master IMU/State ==
  q : Inport
  qd : Inport  Port=2
  q^ : Inport  Port=3
  Master State : Scope  NumInputPorts=2
  Mux : Mux  Inputs=3
  Mux1 : Mux  Inputs=3
  qm : Demux  Outputs=dh.dof
  qm1 : Demux  Outputs=dh.dof
  qs : Demux  Outputs=dh.dof
  wires:
  q/1 -> qm/1
  qd/1 -> qs/1
  qm/1 -> Mux/1
  qs/1 -> Mux/2
  qm/2 -> Mux1/1
  qs/2 -> Mux1/2
  Mux/1 -> Master State/1
  Mux1/1 -> Master State/2
  qm1/2 -> Mux1/3
  q^/1 -> qm1/1
  qm1/1 -> Mux/3

== system Teleoperation_Task_Space/Master IMU/Velocity ==
  dq : Inport
  dqd : Inport  Port=2
  dq^ : Inport  Port=3
  Master Velocity : Scope  NumInputPorts=2
  Mux : Mux  Inputs=3
  Mux1 : Mux  Inputs=3
  qm : Demux  Outputs=dh.dof
  qm1 : Demux  Outputs=dh.dof
  qs : Demux  Outputs=dh.dof
  wires:
  dq/1 -> qm/1
  dqd/1 -> qs/1
  qm/1 -> Mux/1
  qs/1 -> Mux/2
  qm/2 -> Mux1/1
  qs/2 -> Mux1/2
  Mux/1 -> Master Velocity/1
  Mux1/1 -> Master Velocity/2
  qm1/2 -> Mux1/3
  dq^/1 -> qm1/1
  qm1/1 -> Mux/3

== system Teleoperation_Task_Space/Master Observer and Force Estimator/Filter ==
  in : Inport
  Demux : Demux  Outputs=2
  Filter : TransferFcn  Numerator=zdq_B  Denominator=zdq_A
  Filter1 : TransferFcn  Numerator=zdq_B  Denominator=zdq_A
  Mux : Mux  Inputs=2
  out : Outport
  wires:
  Demux/2 -> Filter1/1
  Demux/1 -> Filter/1
  in/1 -> Demux/1
  Mux/1 -> out/1
  Filter/1 -> Mux/1
  Filter1/1 -> Mux/2

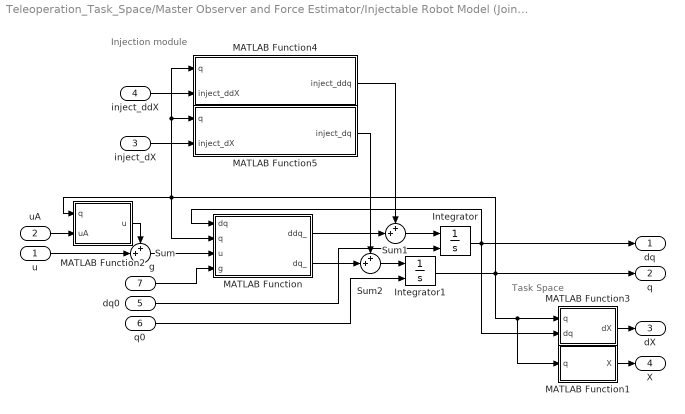
== system Teleoperation_Task_Space/Master Observer and Force Estimator/Injectable Robot Model (Joint Space) ==
  note: Injection module
  note: Task Space
  u : Inport
  uA : Inport  Port=2
  inject_dX : Inport  Port=3
  inject_ddX : Inport  Port=4
  dq0 : Inport  Port=5
  q0 : Inport  Port=6
  g : Inport  Port=7
  Integrator : Integrator  InitialConditionSource=external  InitialCondition=x0
  Integrator1 : Integrator  InitialConditionSource=external  InitialCondition=x0
  MATLAB Function : MATLAB Function  TreatAsAtomicUnit=on
  MATLAB Function1 : MATLAB Function  TreatAsAtomicUnit=on
  MATLAB Function2 : MATLAB Function  TreatAsAtomicUnit=on
  MATLAB Function3 : MATLAB Function  TreatAsAtomicUnit=on
  MATLAB Function4 : MATLAB Function  TreatAsAtomicUnit=on
  MATLAB Function5 : MATLAB Function  TreatAsAtomicUnit=on
  Sum : Sum  Inputs=++|
  Sum1 : Sum  Inputs=++|
  Sum2 : Sum  Inputs=++|
  dq : Outport
  q : Outport  Port=2
  dX : Outport  Port=3
  X : Outport  Port=4
  wires:
  g/1 -> MATLAB Function/4(g)
  u/1 -> Sum/2
  dq0/1 -> Integrator/2
  Integrator1/1 -> q/1, MATLAB Function1/1(q), MATLAB Function3/1(q), MATLAB Function/2(q), MATLAB Function4/1(q), MATLAB Function5/1(q), MATLAB Function2/1(q)
  uA/1 -> MATLAB Function2/2(uA)
  MATLAB Function1/1(X) -> X/1
  Integrator/1 -> dq/1, MATLAB Function3/2(dq), MATLAB Function/1(dq)
  MATLAB Function3/1(dX) -> dX/1
  MATLAB Function2/1(u) -> Sum/1
  Sum/1 -> MATLAB Function/3(u)
  MATLAB Function/1(ddq_) -> Sum1/2
  q0/1 -> Integrator1/2
  Sum1/1 -> Integrator/1
  MATLAB Function/2(dq_) -> Sum2/2
  Sum2/1 -> Integrator1/1
  inject_ddX/1 -> MATLAB Function4/2(inject_ddX)
  inject_dX/1 -> MATLAB Function5/2(inject_dX)
  MATLAB Function4/1(inject_ddq) -> Sum1/1
  MATLAB Function5/1(inject_dq) -> Sum2/1

== system Teleoperation_Task_Space/Master Observer and Force Estimator/Sliding Mode Control ==
  X : Inport
  X_real : Inport  Port=2
  lambdas : Inport  Port=3
  alphas : Inport  Port=4
  Abs : Abs
  Matrix Multiply : Product  Inputs=***
  Matrix Multiply1 : Product
  Sign : Signum
  Sqrt : Sqrt  SaturateOnIntegerOverflow=on
  Sum : Sum  Inputs=-+|
  zm1 : Outport
  zm2 : Outport  Port=2
  wires:
  Sum/1 -> Sign/1, Abs/1
  Abs/1 -> Sqrt/1
  X/1 -> Sum/1
  lambdas/1 -> Matrix Multiply/3
  Sqrt/1 -> Matrix Multiply/2
  X_real/1 -> Sum/2
  Matrix Multiply/1 -> zm1/1  "zm1"
  Matrix Multiply1/1 -> zm2/1  "zm2"
  alphas/1 -> Matrix Multiply1/2
  Sign/1 -> Matrix Multiply/1, Matrix Multiply1/1

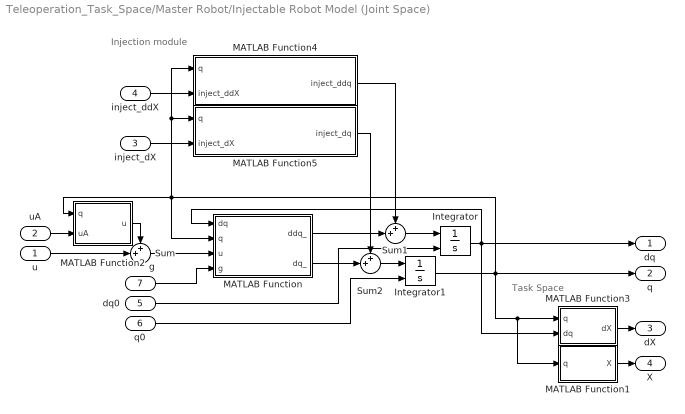
== system Teleoperation_Task_Space/Master Robot/Injectable Robot Model (Joint Space) ==
  note: Injection module
  note: Task Space
  u : Inport
  uA : Inport  Port=2
  inject_dX : Inport  Port=3
  inject_ddX : Inport  Port=4
  dq0 : Inport  Port=5
  q0 : Inport  Port=6
  g : Inport  Port=7
  Integrator : Integrator  InitialConditionSource=external  InitialCondition=x0
  Integrator1 : Integrator  InitialConditionSource=external  InitialCondition=x0
  MATLAB Function : MATLAB Function  TreatAsAtomicUnit=on
  MATLAB Function1 : MATLAB Function  TreatAsAtomicUnit=on
  MATLAB Function2 : MATLAB Function  TreatAsAtomicUnit=on
  MATLAB Function3 : MATLAB Function  TreatAsAtomicUnit=on
  MATLAB Function4 : MATLAB Function  TreatAsAtomicUnit=on
  MATLAB Function5 : MATLAB Function  TreatAsAtomicUnit=on
  Sum : Sum  Inputs=++|
  Sum1 : Sum  Inputs=++|
  Sum2 : Sum  Inputs=++|
  dq : Outport
  q : Outport  Port=2
  dX : Outport  Port=3
  X : Outport  Port=4
  wires:
  g/1 -> MATLAB Function/4(g)
  u/1 -> Sum/2
  dq0/1 -> Integrator/2
  Integrator1/1 -> q/1, MATLAB Function1/1(q), MATLAB Function3/1(q), MATLAB Function/2(q), MATLAB Function4/1(q), MATLAB Function5/1(q), MATLAB Function2/1(q)
  uA/1 -> MATLAB Function2/2(uA)
  MATLAB Function1/1(X) -> X/1
  Integrator/1 -> dq/1, MATLAB Function3/2(dq), MATLAB Function/1(dq)
  MATLAB Function3/1(dX) -> dX/1
  MATLAB Function2/1(u) -> Sum/1
  Sum/1 -> MATLAB Function/3(u)
  MATLAB Function/1(ddq_) -> Sum1/2
  q0/1 -> Integrator1/2
  Sum1/1 -> Integrator/1
  MATLAB Function/2(dq_) -> Sum2/2
  Sum2/1 -> Integrator1/1
  inject_ddX/1 -> MATLAB Function4/2(inject_ddX)
  inject_dX/1 -> MATLAB Function5/2(inject_dX)
  MATLAB Function4/1(inject_ddq) -> Sum1/1
  MATLAB Function5/1(inject_dq) -> Sum2/1

== system Teleoperation_Task_Space/Slave IMU/External Forces ==
  F : Inport
  F^ : Inport  Port=2
  Mux : Mux  Inputs=2
  Mux1 : Mux  Inputs=2
  Slave Fe : Scope  NumInputPorts=2
  qm : Demux  Outputs=dh.dof
  qs : Demux  Outputs=dh.dof
  wires:
  F/1 -> qm/1
  F^/1 -> qs/1
  qm/1 -> Mux/1
  qs/1 -> Mux/2
  qm/2 -> Mux1/1
  qs/2 -> Mux1/2
  Mux/1 -> Slave Fe/1
  Mux1/1 -> Slave Fe/2

== system Teleoperation_Task_Space/Slave IMU/Pose ==
  X : Inport
  X^ : Inport  Port=2
  Mux : Mux  Inputs=2
  Mux1 : Mux  Inputs=2
  Slave Pose : Scope  NumInputPorts=2
  qm : Demux  Outputs=dh.dof
  qm1 : Demux  Outputs=dh.dof
  wires:
  X/1 -> qm/1
  qm/1 -> Mux/1
  qm/2 -> Mux1/1
  Mux/1 -> Slave Pose/1
  Mux1/1 -> Slave Pose/2
  qm1/2 -> Mux1/2
  X^/1 -> qm1/1
  qm1/1 -> Mux/2

== system Teleoperation_Task_Space/Slave IMU/Speed ==
  dX : Inport
  dX^ : Inport  Port=2
  Mux : Mux  Inputs=2
  Mux1 : Mux  Inputs=2
  Slave Speed : Scope  NumInputPorts=2
  qm : Demux  Outputs=dh.dof
  qm1 : Demux  Outputs=dh.dof
  wires:
  dX/1 -> qm/1
  qm/1 -> Mux/1
  qm/2 -> Mux1/1
  Mux/1 -> Slave Speed/1
  Mux1/1 -> Slave Speed/2
  qm1/2 -> Mux1/2
  dX^/1 -> qm1/1
  qm1/1 -> Mux/2

== system Teleoperation_Task_Space/Slave IMU/State ==
  q : Inport
  qd : Inport  Port=2
  q^ : Inport  Port=3
  Mux : Mux  Inputs=3
  Mux1 : Mux  Inputs=3
  Slave State : Scope  NumInputPorts=2
  qm : Demux  Outputs=dh.dof
  qm1 : Demux  Outputs=dh.dof
  qs : Demux  Outputs=dh.dof
  wires:
  q/1 -> qm/1
  qd/1 -> qs/1
  qm/1 -> Mux/1
  qs/1 -> Mux/2
  qm/2 -> Mux1/1
  qs/2 -> Mux1/2
  Mux/1 -> Slave State/1
  Mux1/1 -> Slave State/2
  qm1/2 -> Mux1/3
  q^/1 -> qm1/1
  qm1/1 -> Mux/3

== system Teleoperation_Task_Space/Slave IMU/Velocity ==
  dq : Inport
  dqd : Inport  Port=2
  dq^ : Inport  Port=3
  Mux : Mux  Inputs=3
  Mux1 : Mux  Inputs=3
  Slave Velocity : Scope  NumInputPorts=2
  qm : Demux  Outputs=dh.dof
  qm1 : Demux  Outputs=dh.dof
  qs : Demux  Outputs=dh.dof
  wires:
  dq/1 -> qm/1
  dqd/1 -> qs/1
  qm/1 -> Mux/1
  qs/1 -> Mux/2
  qm/2 -> Mux1/1
  qs/2 -> Mux1/2
  Mux/1 -> Slave Velocity/1
  Mux1/1 -> Slave Velocity/2
  qm1/2 -> Mux1/3
  dq^/1 -> qm1/1
  qm1/1 -> Mux/3

== system Teleoperation_Task_Space/Slave Observer and Force Estimator/Filter ==
  in : Inport
  Demux : Demux  Outputs=2
  Filter : TransferFcn  Numerator=zdq_B  Denominator=zdq_A
  Filter1 : TransferFcn  Numerator=zdq_B  Denominator=zdq_A
  Mux : Mux  Inputs=2
  out : Outport
  wires:
  Demux/2 -> Filter1/1
  Demux/1 -> Filter/1
  in/1 -> Demux/1
  Mux/1 -> out/1
  Filter/1 -> Mux/1
  Filter1/1 -> Mux/2

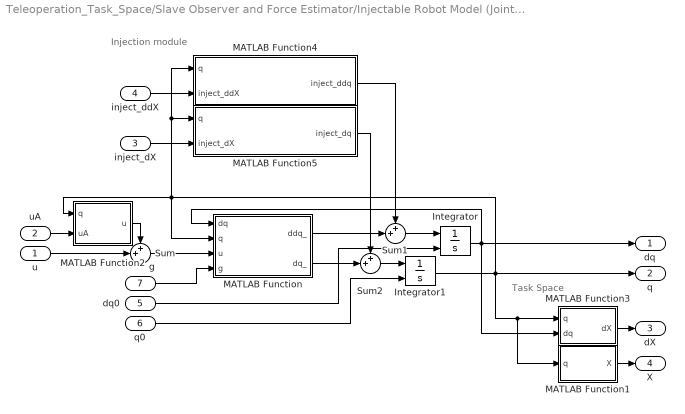
== system Teleoperation_Task_Space/Slave Observer and Force Estimator/Injectable Robot Model (Joint Space) ==
  note: Injection module
  note: Task Space
  u : Inport
  uA : Inport  Port=2
  inject_dX : Inport  Port=3
  inject_ddX : Inport  Port=4
  dq0 : Inport  Port=5
  q0 : Inport  Port=6
  g : Inport  Port=7
  Integrator : Integrator  InitialConditionSource=external  InitialCondition=x0
  Integrator1 : Integrator  InitialConditionSource=external  InitialCondition=x0
  MATLAB Function : MATLAB Function  TreatAsAtomicUnit=on
  MATLAB Function1 : MATLAB Function  TreatAsAtomicUnit=on
  MATLAB Function2 : MATLAB Function  TreatAsAtomicUnit=on
  MATLAB Function3 : MATLAB Function  TreatAsAtomicUnit=on
  MATLAB Function4 : MATLAB Function  TreatAsAtomicUnit=on
  MATLAB Function5 : MATLAB Function  TreatAsAtomicUnit=on
  Sum : Sum  Inputs=++|
  Sum1 : Sum  Inputs=++|
  Sum2 : Sum  Inputs=++|
  dq : Outport
  q : Outport  Port=2
  dX : Outport  Port=3
  X : Outport  Port=4
  wires:
  g/1 -> MATLAB Function/4(g)
  u/1 -> Sum/2
  dq0/1 -> Integrator/2
  Integrator1/1 -> q/1, MATLAB Function1/1(q), MATLAB Function3/1(q), MATLAB Function/2(q), MATLAB Function4/1(q), MATLAB Function5/1(q), MATLAB Function2/1(q)
  uA/1 -> MATLAB Function2/2(uA)
  MATLAB Function1/1(X) -> X/1
  Integrator/1 -> dq/1, MATLAB Function3/2(dq), MATLAB Function/1(dq)
  MATLAB Function3/1(dX) -> dX/1
  MATLAB Function2/1(u) -> Sum/1
  Sum/1 -> MATLAB Function/3(u)
  MATLAB Function/1(ddq_) -> Sum1/2
  q0/1 -> Integrator1/2
  Sum1/1 -> Integrator/1
  MATLAB Function/2(dq_) -> Sum2/2
  Sum2/1 -> Integrator1/1
  inject_ddX/1 -> MATLAB Function4/2(inject_ddX)
  inject_dX/1 -> MATLAB Function5/2(inject_dX)
  MATLAB Function4/1(inject_ddq) -> Sum1/1
  MATLAB Function5/1(inject_dq) -> Sum2/1

== system Teleoperation_Task_Space/Slave Observer and Force Estimator/Sliding Mode Control ==
  X : Inport
  X_real : Inport  Port=2
  lambdas : Inport  Port=3
  alphas : Inport  Port=4
  Abs : Abs
  Matrix Multiply : Product  Inputs=***
  Matrix Multiply1 : Product
  Sign : Signum
  Sqrt : Sqrt  SaturateOnIntegerOverflow=on
  Sum : Sum  Inputs=-+|
  zs1 : Outport
  zs2 : Outport  Port=2
  wires:
  Sum/1 -> Sign/1, Abs/1
  Abs/1 -> Sqrt/1
  X/1 -> Sum/1
  lambdas/1 -> Matrix Multiply/3
  Sqrt/1 -> Matrix Multiply/2
  X_real/1 -> Sum/2
  Matrix Multiply/1 -> zs1/1  "zm1"
  Matrix Multiply1/1 -> zs2/1  "zm2"
  alphas/1 -> Matrix Multiply1/2
  Sign/1 -> Matrix Multiply/1, Matrix Multiply1/1

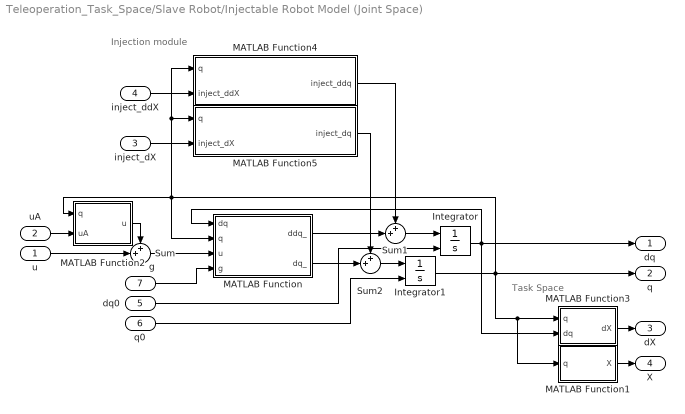
== system Teleoperation_Task_Space/Slave Robot/Injectable Robot Model (Joint Space) ==
  note: Injection module
  note: Task Space
  u : Inport
  uA : Inport  Port=2
  inject_dX : Inport  Port=3
  inject_ddX : Inport  Port=4
  dq0 : Inport  Port=5
  q0 : Inport  Port=6
  g : Inport  Port=7
  Integrator : Integrator  InitialConditionSource=external  InitialCondition=x0
  Integrator1 : Integrator  InitialConditionSource=external  InitialCondition=x0
  MATLAB Function : MATLAB Function  TreatAsAtomicUnit=on
  MATLAB Function1 : MATLAB Function  TreatAsAtomicUnit=on
  MATLAB Function2 : MATLAB Function  TreatAsAtomicUnit=on
  MATLAB Function3 : MATLAB Function  TreatAsAtomicUnit=on
  MATLAB Function4 : MATLAB Function  TreatAsAtomicUnit=on
  MATLAB Function5 : MATLAB Function  TreatAsAtomicUnit=on
  Sum : Sum  Inputs=++|
  Sum1 : Sum  Inputs=++|
  Sum2 : Sum  Inputs=++|
  dq : Outport
  q : Outport  Port=2
  dX : Outport  Port=3
  X : Outport  Port=4
  wires:
  g/1 -> MATLAB Function/4(g)
  u/1 -> Sum/2
  dq0/1 -> Integrator/2
  Integrator1/1 -> q/1, MATLAB Function1/1(q), MATLAB Function3/1(q), MATLAB Function/2(q), MATLAB Function4/1(q), MATLAB Function5/1(q), MATLAB Function2/1(q)
  uA/1 -> MATLAB Function2/2(uA)
  MATLAB Function1/1(X) -> X/1
  Integrator/1 -> dq/1, MATLAB Function3/2(dq), MATLAB Function/1(dq)
  MATLAB Function3/1(dX) -> dX/1
  MATLAB Function2/1(u) -> Sum/1
  Sum/1 -> MATLAB Function/3(u)
  MATLAB Function/1(ddq_) -> Sum1/2
  q0/1 -> Integrator1/2
  Sum1/1 -> Integrator/1
  MATLAB Function/2(dq_) -> Sum2/2
  Sum2/1 -> Integrator1/1
  inject_ddX/1 -> MATLAB Function4/2(inject_ddX)
  inject_dX/1 -> MATLAB Function5/2(inject_dX)
  MATLAB Function4/1(inject_ddq) -> Sum1/1
  MATLAB Function5/1(inject_dq) -> Sum2/1

== system Teleoperation_Task_Space/Slave controller/Sliding Surface ==
  e : Inport
  de : Inport  Port=2
  f : Inport  Port=3
  Integrator : Integrator
  Multiply1 : Gain  Gain=B_s  Multiplication=Matrix(K*u)
  Multiply2 : Gain  Gain=K_s  Multiplication=Matrix(K*u)
  Multiply3 : Gain  Gain=inv(M_s)  Multiplication=Matrix(K*u)
  Sum : Sum  Inputs=|++
  Sum2 : Sum  Inputs=+++
  s : Outport
  wires:
  Multiply3/1 -> Integrator/1
  Integrator/1 -> Sum/1
  Sum2/1 -> Multiply3/1
  f/1 -> Sum2/1
  e/1 -> Multiply2/1
  Multiply2/1 -> Sum2/2
  de/1 -> Sum/2, Multiply1/1
  Multiply1/1 -> Sum2/3
  Sum/1 -> s/1

== system Teleoperation_Task_Space/Slave controller/Subsystem1 ==
  s : Inport
  Abs : Abs
  Constant : Constant  Value=10e-2
  Constant1 : Constant  Value=[1 1]
  Constant2 : Constant
  Divide : Product  Inputs=*/
  Product : Product
  Product1 : Product
  Relational Operator : RelationalOperator  Operator=>  OutDataTypeStr=boolean  RndMeth=Simplest
  Sign : Signum
  Sum : Sum  Inputs=|-+
  Sum1 : Sum  Inputs=+|+
  sat_x : Outport
  wires:
  Divide/1 -> Product1/2, Sign/1, Abs/1
  s/1 -> Divide/1
  Constant/1 -> Divide/2
  Abs/1 -> Relational Operator/1
  Sum1/1 -> sat_x/1
  Sign/1 -> Product/1
  Constant1/1 -> Relational Operator/2
  Relational Operator/1 -> Product/2, Sum/1
  Constant2/1 -> Sum/2
  Sum/1 -> Product1/1
  Product/1 -> Sum1/1
  Product1/1 -> Sum1/2

== matlab function Teleoperation_Task_Space/Master Robot/Injectable Robot Model (Joint Space)/MATLAB Function1 ==
  data: X output; q input; dh parameter
function X = K(q, dh)
    X = K_rne(dh, q);
end

== matlab function Teleoperation_Task_Space/MATLAB Function1 ==
  data: he output; X input; hA input
function he = TAT_1(X, hA)
    TA_ = TA(X);
    rpinv = (TA_*TA_') \ TA_;
    he = rpinv * hA;
end

== matlab function Teleoperation_Task_Space/Master Robot/Injectable Robot Model (Joint Space)/MATLAB Function2 ==
  data: q input; uA input; u output; dh parameter
function u = JAT(q,uA, dh)
    u = JA_rne(dh,q)' * uA;
end

== matlab function Teleoperation_Task_Space/Master Robot/Injectable Robot Model (Joint Space)/MATLAB Function3 ==
  data: dh parameter; dX output; q input; dq input
function dX = JA(dh, q, dq)
    dX = JA_rne(dh, q)*dq;
end

== matlab function Teleoperation_Task_Space/Master Controller/Master Controller ==
  data: dh parameter; qm input size=dh.dof; dqm input size=dh.dof; Xm input size=2; Fm output size=2; dXm input size=2; Fh input size=2; Fe_d input size=2; gravity parameter size=3; M_m parameter size=[2,2]; B_m parameter size=[2,2]; K_m parameter size=[2,2]
function Fm = Cm(dh,qm,dqm, Xm,dXm, Fh,Fe_d,gravity, M_m,B_m,K_m)
    
    BA = BA_rne(dh, qm);
    CAdX = CAdX_rne(dh, qm, dqm);  % we can use CAdX instead of CA*dX since here dq and dX have the same meaning
    GA = GA_rne(dh, qm, gravity);

    % inner impedance controller
    vm = M_m \ (-B_m*dXm - K_m*Xm + Fh - Fe_d);
    % outer decoupling/linearization controller
    Fm = BA*vm + CAdX + GA - Fh;
end

== matlab function Teleoperation_Task_Space/Master Robot/Injectable Robot Model (Joint Space)/MATLAB Function4 ==
  data: q input size=dh.dof; inject_ddq output size=dh.dof; inject_ddX input size=2; dh parameter
function inject_ddq = get_inject_ddq(q, inject_ddX, dh)
    JA = JA_rne(dh, q);
    inject_ddq = pinv(JA) * inject_ddX;
end

== matlab function Teleoperation_Task_Space/Master Robot/Injectable Robot Model (Joint Space)/MATLAB Function5 ==
  data: q input size=dh.dof; inject_dq output size=dh.dof; inject_dX input size=2; dh parameter
function inject_dq = get_inject_dq(q, inject_dX, dh)
    JA = JA_rne(dh, q);
    inject_dq = pinv(JA) * inject_dX;
end

== matlab function Teleoperation_Task_Space/Master Observer and Force Estimator/Injectable Robot Model (Joint Space)/MATLAB Function ==
  data ddq_ settings: updateMethod=SF_CONTINUOUS_TIME_DATA
  data dq_ settings: updateMethod=SF_CONTINUOUS_TIME_DATA
  data dq settings: updateMethod=SF_CONTINUOUS_TIME_DATA
  data q settings: updateMethod=SF_CONTINUOUS_TIME_DATA
  data u settings: updateMethod=SF_CONTINUOUS_TIME_DATA
  data: ddq_ output size=dh.dof; dq_ output size=dh.dof; dq input size=dh.dof; q input size=dh.dof; u input size=dh.dof; g input size=3; dh parameter
function [ddq_, dq_]  = RobotSystem(dq, q, u, g, dh)
    
    % compute dynamics
    B = B_rne(dh, q);
    C = C_rne(dh, q, dq);
    G = G_rne(dh, q, g);

    dq_ = dq(1:dh.dof);

    ddq = B \ (u - C*dq - G);
    ddq_ = ddq(1:dh.dof);
end

== matlab function Teleoperation_Task_Space/Master Observer and Force Estimator/Injectable Robot Model (Joint Space)/MATLAB Function1 ==
  data: X output; q input; dh parameter
function X = K(q, dh)
    X = K_rne(dh, q);
end

== matlab function Teleoperation_Task_Space/Slave Robot/Injectable Robot Model (Joint Space)/MATLAB Function1 ==
  data: X output; q input; dh parameter
function X = K(q, dh)
    X = K_rne(dh, q);
end

== matlab function Teleoperation_Task_Space/Master Observer and Force Estimator/Injectable Robot Model (Joint Space)/MATLAB Function2 ==
  data: q input size=dh.dof; uA input size=2; u output size=dh.dof; dh parameter
function u = JAT(q,uA, dh)
    u = JA_rne(dh,q)' * uA;
end

== matlab function Teleoperation_Task_Space/Master Observer and Force Estimator/Injectable Robot Model (Joint Space)/MATLAB Function3 ==
  data: dh parameter; dX output; q input; dq input
function dX = JA(dh, q, dq)
    dX = JA_rne(dh, q)*dq;
end

== matlab function Teleoperation_Task_Space/Master Observer and Force Estimator/Injectable Robot Model (Joint Space)/MATLAB Function4 ==
  data: q input size=dh.dof; inject_ddq output size=dh.dof; inject_ddX input size=2; dh parameter
function inject_ddq = get_inject_ddq(q, inject_ddX, dh)
    JA = JA_rne(dh, q);
    inject_ddq = pinv(JA) * inject_ddX;
end

== matlab function Teleoperation_Task_Space/Master Observer and Force Estimator/MATLAB Function1 ==
  data: Fh output; q input; zm2eq input; dh parameter
function Fh = BA_zm(q, zm2eq, dh)
     BA = BA_rne(dh, q);
     Fh = BA * zm2eq;
end

== matlab function Teleoperation_Task_Space/Slave Robot/Injectable Robot Model (Joint Space)/MATLAB Function2 ==
  data: q input; uA input; u output; dh parameter
function u = JAT(q,uA, dh)
    u = JA_rne(dh,q)' * uA;
end

== matlab function Teleoperation_Task_Space/Slave Robot/Injectable Robot Model (Joint Space)/MATLAB Function3 ==
  data: dh parameter; dX output; q input; dq input
function dX = JA(dh, q, dq)
    dX = JA_rne(dh, q)*dq;
end

== matlab function Teleoperation_Task_Space/Slave Robot/Injectable Robot Model (Joint Space)/MATLAB Function4 ==
  data: q input size=dh.dof; inject_ddq output size=dh.dof; inject_ddX input size=2; dh parameter
function inject_ddq = get_inject_ddq(q, inject_ddX, dh)
    JA = JA_rne(dh, q);
    inject_ddq = pinv(JA) * inject_ddX;
end

== matlab function Teleoperation_Task_Space/Master Observer and Force Estimator/Injectable Robot Model (Joint Space)/MATLAB Function5 ==
  data: q input size=dh.dof; inject_dq output size=dh.dof; inject_dX input size=2; dh parameter
function inject_dq = get_inject_dq(q, inject_dX, dh)
    JA = JA_rne(dh, q);
    inject_dq = pinv(JA) * inject_dX;
end

== matlab function Teleoperation_Task_Space/Slave Robot/Injectable Robot Model (Joint Space)/MATLAB Function5 ==
  data: q input size=dh.dof; inject_dq output size=dh.dof; inject_dX input size=2; dh parameter
function inject_dq = get_inject_dq(q, inject_dX, dh)
    JA = JA_rne(dh, q);
    inject_dq = pinv(JA) * inject_dX;
end

== matlab function Teleoperation_Task_Space/Slave Observer and Force Estimator/Injectable Robot Model (Joint Space)/MATLAB Function2 ==
  data: q input size=dh.dof; uA input size=2; u output size=dh.dof; dh parameter
function u = JAT(q,uA, dh)
    u = JA_rne(dh,q)' * uA;
end

== matlab function Teleoperation_Task_Space/Slave Robot/Injectable Robot Model (Joint Space)/MATLAB Function ==
  data ddq_ settings: updateMethod=SF_CONTINUOUS_TIME_DATA
  data dq_ settings: updateMethod=SF_CONTINUOUS_TIME_DATA
  data dq settings: updateMethod=SF_CONTINUOUS_TIME_DATA
  data q settings: updateMethod=SF_CONTINUOUS_TIME_DATA
  data u settings: updateMethod=SF_CONTINUOUS_TIME_DATA
  data: ddq_ output size=dh.dof; dq_ output size=dh.dof; dq input size=dh.dof; q input size=dh.dof; u input size=dh.dof; g input size=3; dh parameter
function [ddq_, dq_]  = RobotSystem(dq, q, u, g, dh)
    
    % compute dynamics
    B = B_rne(dh, q);
    C = C_rne(dh, q, dq);
    G = G_rne(dh, q, g);

    dq_ = dq(1:dh.dof);

    ddq = B \ (u - C*dq - G);
    ddq_ = ddq(1:dh.dof);
end
